simulink model "tp3ejercicio5"  (R2021a)
settings: Solver=VariableStepAuto  StartTime=0.0  StopTime=1  RelTol=1e-3
values from neighbouring files (symbols this model uses):
  C = 3  6  9 12 15    [tp1.m]    (also in tp3.m = FaC(F))
undefined symbols (not defined in the file or in its folder): gray, none, Rec, SDTV, videoinput
libraries: visionconversions x1, imaqlib x1
settings Model: Creator=ZeK005  LastModifiedBy=ZeK005

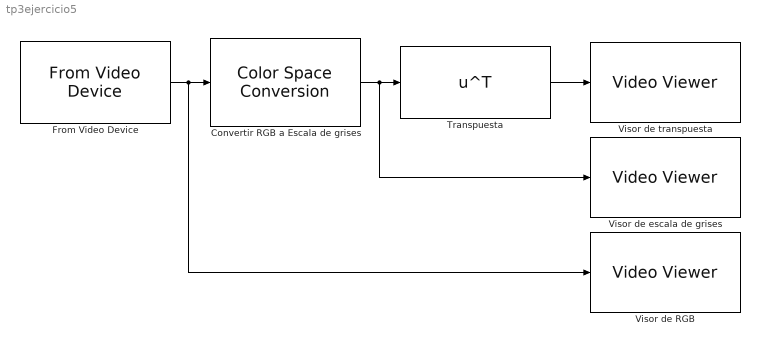
== system tp3ejercicio5 ==
  Convertir RGB a Escala de grises : visionconversions/Color Space  Conversion  conversion=Obsolete  conversionActive=R'G'B' to intensity  wp_str=D65  rec=Rec. 601 (SDTV)  sys=1125/60/2:1  imagePorts=One multidimensional signal
  From Video Device : imaqlib/From Video Device  DeviceMenu=winvideo 2 (OBS Virtual Camera)  Device=winvideo 2 (OBS Virtual Camera)  ObjConstructor=videoinput('winvideo', 2)  VideoFormatMenu=I420_640x360  VideoFormat=I420_640x360  VideoSource=input1  ROIPosition=[0 0 360 640]  EnableHWTrigger=off  TriggerConfiguration=none/none  SampleTime=1/30  OutputPortsMode=One multidimensional signal  DataType=single  CanDoHWTrigger=no  ReturnedColorSpace=rgb  BlockHandle=1851.0001  ROIWidth=640  ROIHeight=360  ROIColumn=0  ROIRow=0  EngXMLPath=C:\Program Files\Polyspace\R2021a\toolbox\imaq\imaq\private  DevXMLPath=C:\ProgramData\MATLAB\SupportPackages\R2021a\toolbox\imaq\supportpackages\genericvideo\adaptor\win64  EngLibPath=C:\Program Files\Polyspace\R2021a\toolbox\imaq\imaqblks\imaqmex\win64  ColorSpace=rgb  BayerSensorAlignment=grbg  ImaqMode=off
  Transpuesta : Math  Operator=transpose  SaturateOnIntegerOverflow=on
  Visor de RGB : VideoViewer  FigPos=[277 511 638 399]
  Visor de escala de grises : VideoViewer  colormapValue=gray(256)  FigPos=[277 1022 638 400]
  Visor de transpuesta : VideoViewer  colormapValue=gray(256)  FigPos=[916 1020 503 908]
  wires:
  From Video Device/1 -> Visor de RGB/1, Convertir RGB a Escala de grises/1
  Convertir RGB a Escala de grises/1 -> Visor de escala de grises/1, Transpuesta/1
  Transpuesta/1 -> Visor de transpuesta/1
